simulink model "inverter_3_phase"  (R2021a)
settings: Solver=ode4  StartTime=0.0  StopTime=0.1  FixedStep=1e-6  RelTol=1e-3
libraries: spsIGBTDiodeLib x6, spsDCVoltageSourceLib x1, spsGroundLib x1, spsThreePhaseSeriesRLCBranchLib x1, spsThreePhaseVIMeasurementLib x1, simulink x1, spspowerguiLib x1
settings Model: Creator=PRANAY KAMAL  LastModifiedBy=PRANAY KAMAL
settings DataIOCC: ReturnWorkspaceOutputs=off

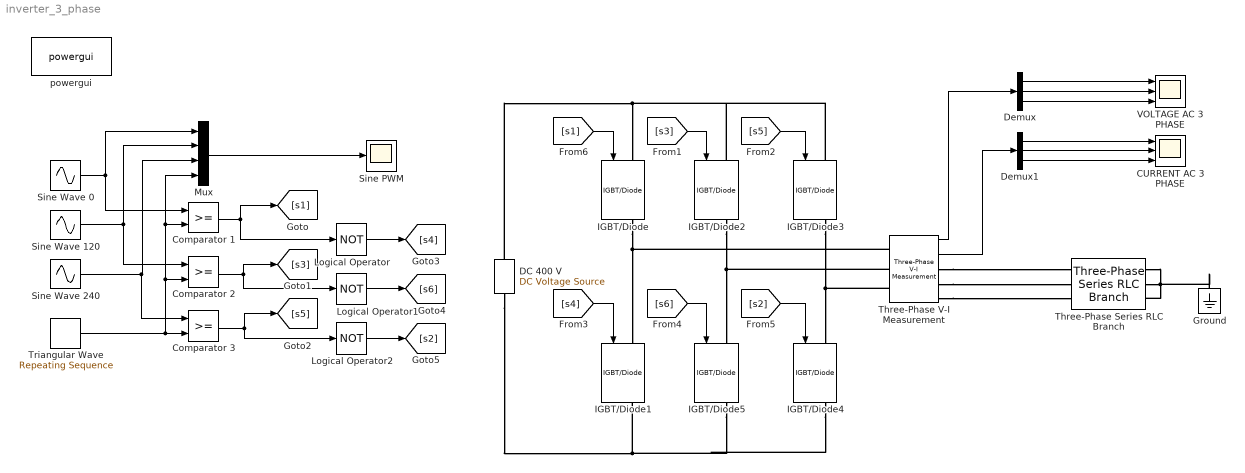
== system inverter_3_phase ==
  CURRENT AC 3 PHASE : Scope  NumInputPorts=3
  Comparator 1 : RelationalOperator  OutDataTypeStr=boolean  RndMeth=Simplest
  Comparator 2 : RelationalOperator  OutDataTypeStr=boolean  RndMeth=Simplest
  Comparator 3 : RelationalOperator  OutDataTypeStr=boolean  RndMeth=Simplest
  DC 400 V : spsDCVoltageSourceLib/DC Voltage Source  Amplitude=400  Measurements=None
  Demux : Demux  Outputs=3
  Demux1 : Demux  Outputs=3
  Ground : spsGroundLib/Ground  LConnTagsString=a
  IGBT/Diode{,1..5} (6 alike) : spsIGBTDiodeLib/IGBT//Diode  Ron=1e-3  Rs=1e5  Cs=inf  Measurements=on
  Logical Operator : Logic  Operator=NOT  AllPortsSameDT=off  OutDataTypeStr=boolean
  Logical Operator1 : Logic  Operator=NOT  AllPortsSameDT=off  OutDataTypeStr=boolean
  Logical Operator2 : Logic  Operator=NOT  AllPortsSameDT=off  OutDataTypeStr=boolean
  Mux : Mux
  Sine PWM : Scope
  Sine Wave 0 : Sin  Amplitude=0.8  Frequency=2*pi*50  SampleTime=0
  Sine Wave 120 : Sin  Amplitude=0.8  Frequency=2*pi*50  Phase=2*pi/3  SampleTime=0
  Sine Wave 240 : Sin  Amplitude=0.8  Frequency=2*pi*50  Phase=-2*pi/3  SampleTime=0
  Three-Phase Series RLC Branch : spsThreePhaseSeriesRLCBranchLib/Three-Phase Series RLC Branch  LConnTagsString=A|B|C  RConnTagsString=A|B|C  BranchType=RL  Resistance=1  Inductance=1e-2  Capacitance=1e-6  Measurements=None
  Three-Phase V-I Measurement : spsThreePhaseVIMeasurementLib/Three-Phase V-I Measurement  VoltageMeasurement=phase-to-ground  SetLabelV=off  LabelV=Vabc  Vpu=off  VpuLL=off  CurrentMeasurement=yes  SetLabelI=off  LabelI=Iabc  Ipu=off  Pbase=100e6  Vbase=500e3  OutputType=Complex  PhasorSimulation=off  PSBequivalent=0
  Triangular Wave : simulink/Sources/Repeating Sequence  rep_seq_t=[0 0.5 1]*[1/6000]  rep_seq_y=[1 -1 1]
  VOLTAGE AC 3 PHASE : Scope  NumInputPorts=3
  powergui : spspowerguiLib/powergui  Priority=1  SimulationMode=Continuous  SampleTime=50e-6  frequency=60  Iterations=50  frequencyindice=0  Pbase=100e6  ErrMax=1e-4  UnitsV=kV  UnitsW=MW  buscounter=0  FunctionMessages=off  echomessages=off  EnableUseOfTLC=off  CurrentSourceSwitches=off  DisableSnubberDevices=off  DisableRonSwitches=off  DisableVfSwitches=off  DisplayEquations=off  AutomaticDiscreteSolvers=off  SolverType=Tustin/Backward Euler (TBE)  Interpol=off  ExternalGateDelay=off  methode=off  Ts=100  x0status=blocks  SPID=on  SwTol=0  HookPort=off  NonlinearTolerance=1e-4  nMaxIteration=100  ContinueOnMaxIteration=off  RestoreLinks=warning  ResistiveCurrentMeasurement=off  Frange=[0:2:500]  Ylog=off  Xlog=on  ShowGrid=off  save=off  variable=ZData  structure=0  ZoomFFT=off  StartTime=0.0  cycles=1  DisplayStyle=1  fundamental=60  FreqAxis=off  MaxFrequency=1000  frequencyindicesteady=1  RmsSteady=1  display=off
  wires:
  Sine Wave 0/1 -> Mux/1, Comparator 1/1
  Sine Wave 120/1 -> Mux/2, Comparator 2/1
  Sine Wave 240/1 -> Comparator 3/1, Mux/3
  Triangular Wave/1 -> Comparator 3/2, Comparator 2/2, Comparator 1/2, Mux/4
  Mux/1 -> Sine PWM/1
  Comparator 1/1 -> Logical Operator/1, [s1]
  Comparator 2/1 -> Logical Operator1/1, [s3]
  Comparator 3/1 -> Logical Operator2/1, [s5]
  Logical Operator/1 -> [s4]
  Logical Operator2/1 -> [s2]
  Logical Operator1/1 -> [s6]
  [s3] -> IGBT/Diode2/1
  [s5] -> IGBT/Diode3/1
  [s4] -> IGBT/Diode1/1
  [s6] -> IGBT/Diode5/1
  [s2] -> IGBT/Diode4/1
  [s1] -> IGBT/Diode/1
  Three-Phase V-I Measurement/1 -> Demux/1
  Demux/1 -> VOLTAGE AC 3 PHASE/1
  Demux/2 -> VOLTAGE AC 3 PHASE/2
  Demux/3 -> VOLTAGE AC 3 PHASE/3
  Demux1/2 -> CURRENT AC 3 PHASE/2
  Three-Phase V-I Measurement/2 -> Demux1/1
  Demux1/1 -> CURRENT AC 3 PHASE/1
  Demux1/3 -> CURRENT AC 3 PHASE/3
  connections:
  DC 400 V/RConn1 -- IGBT/Diode2/LConn1 -- IGBT/Diode3/LConn1 -- IGBT/Diode/LConn1
  DC 400 V/LConn1 -- IGBT/Diode4/RConn1 -- IGBT/Diode5/RConn1 -- IGBT/Diode1/RConn1
  IGBT/Diode/RConn1 -- Three-Phase V-I Measurement/LConn1 -- IGBT/Diode1/LConn1
  IGBT/Diode2/RConn1 -- Three-Phase V-I Measurement/LConn2 -- IGBT/Diode5/LConn1
  IGBT/Diode3/RConn1 -- Three-Phase V-I Measurement/LConn3 -- IGBT/Diode4/LConn1
  Three-Phase V-I Measurement/RConn1 -- Three-Phase Series RLC Branch/LConn1
  Three-Phase V-I Measurement/RConn2 -- Three-Phase Series RLC Branch/LConn2
  Three-Phase V-I Measurement/RConn3 -- Three-Phase Series RLC Branch/LConn3
  Three-Phase Series RLC Branch/RConn1 -- Ground/LConn1 -- Three-Phase Series RLC Branch/RConn2 -- Three-Phase Series RLC Branch/RConn3
